simulink model "wheelsdown_sim"  (R2018b)
settings: Solver=VariableStepAuto  StartTime=0.0  StopTime=10.0  RelTol=1e-3
values from neighbouring files (symbols this model uses):
  K_p = 0.45    [script.m]
settings Model: Creator=megam  LastModifiedBy=megam

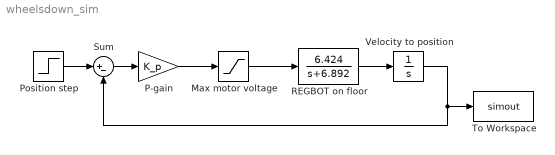
== system wheelsdown_sim ==
  "Max motor voltage " : Saturate  UpperLimit=3  LowerLimit=0
  P-gain : Gain  Gain=K_p
  Position step : Step  Time=0.5  Before=2  After=4  SampleTime=0
  REGBOT on floor : TransferFcn  Numerator=[6.424]  Denominator=[1 6.892]
  Sum : Sum  Inputs=|+-
  To Workspace : ToWorkspace  VariableName=simout  SaveFormat=Timeseries  SampleTime=-1
  Velocity to position : Integrator
  wires:
  Position step/1 -> Sum/1
  Sum/1 -> P-gain/1
  P-gain/1 -> "Max motor voltage "/1
  "Max motor voltage "/1 -> REGBOT on floor/1
  REGBOT on floor/1 -> Velocity to position/1
  Velocity to position/1 -> To Workspace/1, Sum/2
